simulink model "sf_cycle_error_fix"  (Simulink 7.6)
settings: Solver=ode45  StartTime=0.0  StopTime=10.0  RelTol=1e-3
settings Model: Creator=The MathWorks Inc.  CovMetricSettings=dcmtr  ExtModeTrigMode=oneshot  ExtModeArmWhenConnect=off  ExtModeAutoUpdateStatusClock=off
settings DataIOCC: LimitDataPoints=off
settings OptimizationCC: BooleanDataType=off  InlineInvariantSignals=on  InitFltsAndDblsToZero=on
settings DebuggingCC: SaveWithParameterizedLinksMsg=none  SignalResolutionControl=TryResolveAllWithWarning  SolverPrmCheckMsg=none  MultiTaskDSMMsg=warning  MultiTaskCondExecSysMsg=none  StrictBusMsg=None
settings HardwareCC: TargetUnknown=on
settings SFSimCC: SimParseCustomCode=off
settings RTWCC: IncludeERTFirstTime=on
settings GRTTargetCC: TargetFcnLib=ansi_tfl_tmw.mat

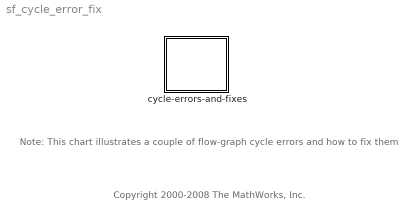
== system sf_cycle_error_fix ==
  note: Note: This chart illustrates a couple of flow-graph
      | cycle errors and  how to fix them
  note: Copyright 2000-2008 The MathWorks, Inc.
  cycle-errors-and-fixes : Stateflow chart  TreatAsAtomicUnit=on

== stateflow chart cycle-errors-and-fixes ==
  state Error1: [group]
    The bottom junction in the loop
    does not have an unconditional
    path to termination
    (default) -> (junction 8)
    (junction 8) -> (junction 9) : {action1;}
    (junction 9) -> (junction 8) [order 2] : [c2]
    (junction 9) -> (junction 10) [order 1] : [c1]
  state Fix1: [group]
    We incorporate the negation of condition c1
    into the transition containing c2 such that the
    resulting diagram is functionally equivalent
    and has an unconditional path out of the loop
    to termination.
    (default) -> (junction 11)
    (junction 12) -> (junction 11) [order 1] : [!c1 && c2]
    (junction 11) -> (junction 12) : {action2;}
    (junction 12) -> (junction 13) [order 2]
  state Error2: [group]
    The top junction in the loop
    does not have an unconditional
    path to termination
    (default) -> (junction 14)
    (junction 15) -> (junction 14) [order 1] : [c2]
    (junction 14) -> (junction 15) : [c1]{action1;}
    (junction 15) -> (junction 16) [order 2] : {action2;}
  state Fix2: [group]
    We create an unconditional transition from
    the top junction to the terminal junction.
    Once again, this is functionally equivalent
    (default) -> (junction 17)
    (junction 18) -> (junction 17) [order 1] : [c2]
    (junction 17) -> (junction 18) [order 1] : [c1]{action1;}
    (junction 18) -> (junction 19) [order 2] : {action2;}
    (junction 17) -> (junction 19) [order 2]
  state Note: [group]
    The following diagrams illustrate a couple of flow-graph cycle errors and  how to fix them
